simulink model "clearing_faulted_segment_travelling_Wave"  (R2018a)
settings: Solver=ode23t  StartTime=0.0  StopTime=2  MaxStep=1e-3  RelTol=1e-3
values from neighbouring files (symbols this model uses):
  AC_lim = [1.5 -1.5]    [MT_HVDC_initialize.m]
  C_pm = 10.48e-3    (= 0.01048)    [MT_HVDC_initialize.m]
  ccsc_lim = [1.0 -1.0]    [MT_HVDC_initialize.m]
  DC_lim = [1.05 -1.05]    [MT_HVDC_initialize.m]
  f = 50    [MT_HVDC_initialize.m]
  Fc = 50    [MT_HVDC_initialize.m]
  Fn_filter = 1000    [MT_HVDC_initialize.m]
  Ireg_lim_i = [1.5, -1.5]    [MT_HVDC_initialize.m]
  Ireg_lim_r = [1.5, -1.5]    [MT_HVDC_initialize.m]
  Ki_ACreg_i = 260    [MT_HVDC_initialize.m]
  Ki_ccsc = 5    [MT_HVDC_initialize.m]
  Ki_DCreg_r = 150    [MT_HVDC_initialize.m]
  Ki_Ireg_i = 200    [MT_HVDC_initialize.m]
  Ki_Ireg_r = 100    [MT_HVDC_initialize.m]
  Ki_R_inv = 150000    [MT_HVDC_initialize.m]
  Ki_R_rec = 5000    [MT_HVDC_initialize.m]
  Kp_ACreg_i = 2    [MT_HVDC_initialize.m]
  Kp_ccsc = 1    [MT_HVDC_initialize.m]
  Kp_DCreg_r = 8    [MT_HVDC_initialize.m]
  Kp_Ireg_i = 2    [MT_HVDC_initialize.m]
  Kp_Ireg_r = 2    [MT_HVDC_initialize.m]
  Kp_R_inv = 0.001    [MT_HVDC_initialize.m]
  Kp_R_rec = 0.001    [MT_HVDC_initialize.m]
  L1_pu = 0.109    [MT_HVDC_initialize.m]
  L2_pu = 0.0824    [MT_HVDC_initialize.m]
  L_arm = L_arm_pu*Z_base66/w    [MT_HVDC_initialize.m]
  L_arm_pu = 0.15    [MT_HVDC_initialize.m]
  L_int = X_int/w    [MT_HVDC_initialize.m]
  n = 50    [MT_HVDC_initialize.m]
  n2 = 50    [MT_HVDC_initialize.m]
  P_nom = 220e6    (= 220000000)    [MT_HVDC_initialize.m]
  R1_pu = 0.00206    [MT_HVDC_initialize.m]
  R2_pu = 0.00206    [MT_HVDC_initialize.m]
  R_arm = 0.03    [MT_HVDC_initialize.m]
  R_arm_pu = R_arm/Z_base66    [MT_HVDC_initialize.m]
  R_int = sqrt((z_int_400^2)/(1+xr_ratio^2))    [MT_HVDC_initialize.m]
  Rg_T1 = 40    [MT_HVDC_initialize.m]
  S1_nom = P_nom    (= 220000000)    [MT_HVDC_initialize.m]
  S2_nom = P_nom    (= 220000000)    [MT_HVDC_initialize.m]
  T_fault = 1.4    [MT_HVDC_initialize.m]
  Ts_Control = 40e-6    (= 4e-05)    [MT_HVDC_initialize.m]
  Ts_Power = 20e-6    (= 2e-05)    [MT_HVDC_initialize.m]
  V1_prim = V_prim    (= 400000)    [MT_HVDC_initialize.m]
  V1_sec = V_grid    (= 66000)    [MT_HVDC_initialize.m]
  V2_prim = V_grid    (= 66000)    [MT_HVDC_initialize.m]
  V2_sec = 18e3    (= 18000)    [MT_HVDC_initialize.m]
  V_ac_ref = 1.035    [MT_HVDC_initialize.m]
  V_grid = 66e3    (= 66000)    [MT_HVDC_initialize.m]
  V_prim = 400e3    (= 400000)    [MT_HVDC_initialize.m]
  Vc_pm_r = 0*Vdc_nom/n    (= 0)    [MT_HVDC_initialize.m]
  Vdc_nom = 135e3    (= 135000)    [MT_HVDC_initialize.m]
  w = 2*pi*f    (= 314.159265359)    [MT_HVDC_initialize.m]
  z0z1 = 0.8    [MT_HVDC_initialize.m]
  Zeta_filter = 1    [MT_HVDC_initialize.m]
undefined symbols (not defined in the file or in its folder): D1, Delta, DiscIntNeverNeededParam
libraries: powerlib x417, powerlib_meascontrol x130, simulink x84, powerlib_extras x8, simulink_extras x5
(part 3 of 17)

== system clearing_faulted_segment_travelling_Wave/MMC Converter1 ==
  g : Inport
  Current Measurement{,1..5} (6 alike) : powerlib/Measurements/Current Measurement  PhasorSimulation=off  OutputType=Complex  PSBequivalent=0
      settings: SourceProductName=Simscape Electrical
  Demux : Demux  Outputs=6
  Half-Bridge MMC Ap : Subsystem  mask(Half-Bridge MMC - Aggregate Model){n=n, C=C_pm, Vc_Initial=Vc_pm_r, Ts=Ts_Power}
      mask prompts: n "Number of power modules"; C "Capacitor value (F):"; Vc_Initial "Capacitor initial voltage (V):"; Ts "Sample time (s):"
      mask help:
      | Implement a half-bridge Modular Multilevel Converter (MMC) using a switching-function model where only one equivalent module is used to represent all power modules.
      |
      | The control signal is a two-element vector [ Nin, Nbl ], where Nin represents the number of inserted modules and Nbl represents the number of modules in the blocked-state. The output Vc (capacitor voltage) has only one element and gives the average value of the capacitors modules.
      |
      | With this aggregate model, it is assumed that capacitor voltage of all power modules are well-balanced. However, control system dynamics, converter harmonics content and circulating currents phenomena are all-well represented. The model runs a lot faster than the detailed model which uses two switching devices and one capacitor for each individual power module. This aggregate model is also well-suited for real-time simulation.
      settings: AttributesFormatString=(Aggregate model of %<n> PM)
      mask Display:
      | x1=0.0;
      | plot([0.17 0.5]+x1,[0.93 0.93])
      | plot([0.5 0.5]+x1,[0.93,0.80])
      | plot([0.5 0.38]+x1,[0.80 0.74])
      | plot([0.38 0.38]+x1,[0.80 0.62])
      | plot([0.38 0.5]+x1,[0.68 0.62])
      | plot([0.5 0.5]+x1,[0.62 0.52])
      | plot([0.45 0.5 0.43]+x1,[0.68 0.62 0.60])
      | %
      | y1=0.40-0.03;
      | plot([0.5 0.5]+x1,[0.93,0.80]-y1)
      | plot([0.5 0.38]+x1,[0.80 0.74]-y1)
      | plot([0.38 0.38]+x1,[0.80 0.62]-y1)
      | plot([0.38 0.5]+x1,[0.68 0.62]-y1)
      | plot([0.5 0.5]+x1,[0.62 0.52]-y1)
      | plot([0.45 0.5 0.43]+x1,[0.68 0.62 0.60]-y1)
      | plot([0.5 0.5]+x1,[0.2,0.10])
      | plot([0.17 0.5]+x1,[0.1 0.1])
      | %
      | plot([0.5 0.6]+x1,[0.84 0.84]+0.03)
      | plot([0.6 0.6]+x1,[0.84 0.74]+0.03)
      | plot([0.6 0.56]+x1,[0.74 0.69]+0.03)
      | plot([0.6 0.64]+x1,[0.74 0.69]+0.03)
      | plot([0.56 0.64]+x1,[0.69 0.69]+0.03)
      | plot([0.6 0.6]+x1,[0.69 0.57]+0.03)
      | plot([0.5 0.6]+x1,[0.57 0.57]+0.03)
      | plot([0.55 0.65]+x1,[0.74 0.74]+0.03)
      | %
      | y2=0.4-0.03;
      | plot([0.5 0.6]+x1,[0.84 0.84]-y2)
      | plot([0.6 0.6]+x1,[0.84 0.74]-y2)
      | plot([0.6 0.56]+x1,[0.74 0.69]-y2)
      | plot([0.6 0.64]+x1,[0.74 0.69]-y2)
      | plot([0.56 0.64]+x1,[0.69 0.69]-y2)
      | plot([0.6 0.6]+x1,[0.69 0.57]-y2)
      | plot([0.5 0.6]+x1,[0.57 0.57]-y2)
      | plot([0.55 0.65]+x1,[0.74 0.74]-y2)
      | %
      | plot([0.5 0.75]+x1,[0.53 0.53])
      | plot([0.75 0.75]+x1,[0.53 0.57])
      | plot([0.75 0.75]+x1,[0.61 0.65])
      | plot([0.75 0.75]+x1,[0.69 0.73])
      | plot([0.75 0.75]+x1,[0.77 0.81])
      | plot([0.75 0.75]+x1,[0.09 0.07])
      | plot([0.75 0.75]+x1,[0.04 0.01])
      | %
      | plot([0.34 0.34]+x1,[0.65 0.75])
      | plot([0.28 0.34]+x1,[0.7 0.7])
      | %
      | plot([0.34 0.34]+x1,[0.65 0.75]-y2)
      | plot([0.28 0.34]+x1,[0.7 0.7]-y2)
      | %
      | %Capacitor
      | plot([0.16 0.16],[0.93 0.54])
      | plot([0.16 0.16],[0.47 0.10])
      | plot([0.04 0.27],[0.54 0.54])
      | plot([0.04 0.27],[0.47 0.47])
      | %
      | plot([0.5 0.75],[0.1 0.1])
      | % text(0.78,0.5,'1')
      | % text(0.78,0.12,'2')
      | %
      | color('blue')
      | port_label('input',1,'N')
  Half-Bridge MMC Ap1 : Subsystem  mask(Half-Bridge MMC - Aggregate Model){n=n, C=C_pm, Vc_Initial=Vc_pm_r, Ts=Ts_Power}
      mask prompts: n "Number of power modules"; C "Capacitor value (F):"; Vc_Initial "Capacitor initial voltage (V):"; Ts "Sample time (s):"
      mask help:
      | Implement a half-bridge Modular Multilevel Converter (MMC) using a switching-function model where only one equivalent module is used to represent all power modules.
      |
      | The control signal is a two-element vector [ Nin, Nbl ], where Nin represents the number of inserted modules and Nbl represents the number of modules in the blocked-state. The output Vc (capacitor voltage) has only one element and gives the average value of the capacitors modules.
      |
      | With this aggregate model, it is assumed that capacitor voltage of all power modules are well-balanced. However, control system dynamics, converter harmonics content and circulating currents phenomena are all-well represented. The model runs a lot faster than the detailed model which uses two switching devices and one capacitor for each individual power module. This aggregate model is also well-suited for real-time simulation.
      settings: AttributesFormatString=(Aggregate model of %<n> PM)
      mask Display:
      | x1=0.0;
      | plot([0.17 0.5]+x1,[0.93 0.93])
      | plot([0.5 0.5]+x1,[0.93,0.80])
      | plot([0.5 0.38]+x1,[0.80 0.74])
      | plot([0.38 0.38]+x1,[0.80 0.62])
      | plot([0.38 0.5]+x1,[0.68 0.62])
      | plot([0.5 0.5]+x1,[0.62 0.52])
      | plot([0.45 0.5 0.43]+x1,[0.68 0.62 0.60])
      | %
      | y1=0.40-0.03;
      | plot([0.5 0.5]+x1,[0.93,0.80]-y1)
      | plot([0.5 0.38]+x1,[0.80 0.74]-y1)
      | plot([0.38 0.38]+x1,[0.80 0.62]-y1)
      | plot([0.38 0.5]+x1,[0.68 0.62]-y1)
      | plot([0.5 0.5]+x1,[0.62 0.52]-y1)
      | plot([0.45 0.5 0.43]+x1,[0.68 0.62 0.60]-y1)
      | plot([0.5 0.5]+x1,[0.2,0.10])
      | plot([0.17 0.5]+x1,[0.1 0.1])
      | %
      | plot([0.5 0.6]+x1,[0.84 0.84]+0.03)
      | plot([0.6 0.6]+x1,[0.84 0.74]+0.03)
      | plot([0.6 0.56]+x1,[0.74 0.69]+0.03)
      | plot([0.6 0.64]+x1,[0.74 0.69]+0.03)
      | plot([0.56 0.64]+x1,[0.69 0.69]+0.03)
      | plot([0.6 0.6]+x1,[0.69 0.57]+0.03)
      | plot([0.5 0.6]+x1,[0.57 0.57]+0.03)
      | plot([0.55 0.65]+x1,[0.74 0.74]+0.03)
      | %
      | y2=0.4-0.03;
      | plot([0.5 0.6]+x1,[0.84 0.84]-y2)
      | plot([0.6 0.6]+x1,[0.84 0.74]-y2)
      | plot([0.6 0.56]+x1,[0.74 0.69]-y2)
      | plot([0.6 0.64]+x1,[0.74 0.69]-y2)
      | plot([0.56 0.64]+x1,[0.69 0.69]-y2)
      | plot([0.6 0.6]+x1,[0.69 0.57]-y2)
      | plot([0.5 0.6]+x1,[0.57 0.57]-y2)
      | plot([0.55 0.65]+x1,[0.74 0.74]-y2)
      | %
      | plot([0.5 0.75]+x1,[0.53 0.53])
      | plot([0.75 0.75]+x1,[0.53 0.57])
      | plot([0.75 0.75]+x1,[0.61 0.65])
      | plot([0.75 0.75]+x1,[0.69 0.73])
      | plot([0.75 0.75]+x1,[0.77 0.81])
      | plot([0.75 0.75]+x1,[0.09 0.07])
      | plot([0.75 0.75]+x1,[0.04 0.01])
      | %
      | plot([0.34 0.34]+x1,[0.65 0.75])
      | plot([0.28 0.34]+x1,[0.7 0.7])
      | %
      | plot([0.34 0.34]+x1,[0.65 0.75]-y2)
      | plot([0.28 0.34]+x1,[0.7 0.7]-y2)
      | %
      | %Capacitor
      | plot([0.16 0.16],[0.93 0.54])
      | plot([0.16 0.16],[0.47 0.10])
      | plot([0.04 0.27],[0.54 0.54])
      | plot([0.04 0.27],[0.47 0.47])
      | %
      | plot([0.5 0.75],[0.1 0.1])
      | % text(0.78,0.5,'1')
      | % text(0.78,0.12,'2')
      | %
      | color('blue')
      | port_label('input',1,'N')
  Half-Bridge MMC Ap2 : Subsystem  mask(Half-Bridge MMC - Aggregate Model){n=n, C=C_pm, Vc_Initial=Vc_pm_r, Ts=Ts_Power}
      mask prompts: n "Number of power modules"; C "Capacitor value (F):"; Vc_Initial "Capacitor initial voltage (V):"; Ts "Sample time (s):"
      mask help:
      | Implement a half-bridge Modular Multilevel Converter (MMC) using a switching-function model where only one equivalent module is used to represent all power modules.
      |
      | The control signal is a two-element vector [ Nin, Nbl ], where Nin represents the number of inserted modules and Nbl represents the number of modules in the blocked-state. The output Vc (capacitor voltage) has only one element and gives the average value of the capacitors modules.
      |
      | With this aggregate model, it is assumed that capacitor voltage of all power modules are well-balanced. However, control system dynamics, converter harmonics content and circulating currents phenomena are all-well represented. The model runs a lot faster than the detailed model which uses two switching devices and one capacitor for each individual power module. This aggregate model is also well-suited for real-time simulation.
      settings: AttributesFormatString=(Aggregate model of %<n> PM)
      mask Display:
      | x1=0.0;
      | plot([0.17 0.5]+x1,[0.93 0.93])
      | plot([0.5 0.5]+x1,[0.93,0.80])
      | plot([0.5 0.38]+x1,[0.80 0.74])
      | plot([0.38 0.38]+x1,[0.80 0.62])
      | plot([0.38 0.5]+x1,[0.68 0.62])
      | plot([0.5 0.5]+x1,[0.62 0.52])
      | plot([0.45 0.5 0.43]+x1,[0.68 0.62 0.60])
      | %
      | y1=0.40-0.03;
      | plot([0.5 0.5]+x1,[0.93,0.80]-y1)
      | plot([0.5 0.38]+x1,[0.80 0.74]-y1)
      | plot([0.38 0.38]+x1,[0.80 0.62]-y1)
      | plot([0.38 0.5]+x1,[0.68 0.62]-y1)
      | plot([0.5 0.5]+x1,[0.62 0.52]-y1)
      | plot([0.45 0.5 0.43]+x1,[0.68 0.62 0.60]-y1)
      | plot([0.5 0.5]+x1,[0.2,0.10])
      | plot([0.17 0.5]+x1,[0.1 0.1])
      | %
      | plot([0.5 0.6]+x1,[0.84 0.84]+0.03)
      | plot([0.6 0.6]+x1,[0.84 0.74]+0.03)
      | plot([0.6 0.56]+x1,[0.74 0.69]+0.03)
      | plot([0.6 0.64]+x1,[0.74 0.69]+0.03)
      | plot([0.56 0.64]+x1,[0.69 0.69]+0.03)
      | plot([0.6 0.6]+x1,[0.69 0.57]+0.03)
      | plot([0.5 0.6]+x1,[0.57 0.57]+0.03)
      | plot([0.55 0.65]+x1,[0.74 0.74]+0.03)
      | %
      | y2=0.4-0.03;
      | plot([0.5 0.6]+x1,[0.84 0.84]-y2)
      | plot([0.6 0.6]+x1,[0.84 0.74]-y2)
      | plot([0.6 0.56]+x1,[0.74 0.69]-y2)
      | plot([0.6 0.64]+x1,[0.74 0.69]-y2)
      | plot([0.56 0.64]+x1,[0.69 0.69]-y2)
      | plot([0.6 0.6]+x1,[0.69 0.57]-y2)
      | plot([0.5 0.6]+x1,[0.57 0.57]-y2)
      | plot([0.55 0.65]+x1,[0.74 0.74]-y2)
      | %
      | plot([0.5 0.75]+x1,[0.53 0.53])
      | plot([0.75 0.75]+x1,[0.53 0.57])
      | plot([0.75 0.75]+x1,[0.61 0.65])
      | plot([0.75 0.75]+x1,[0.69 0.73])
      | plot([0.75 0.75]+x1,[0.77 0.81])
      | plot([0.75 0.75]+x1,[0.09 0.07])
      | plot([0.75 0.75]+x1,[0.04 0.01])
      | %
      | plot([0.34 0.34]+x1,[0.65 0.75])
      | plot([0.28 0.34]+x1,[0.7 0.7])
      | %
      | plot([0.34 0.34]+x1,[0.65 0.75]-y2)
      | plot([0.28 0.34]+x1,[0.7 0.7]-y2)
      | %
      | %Capacitor
      | plot([0.16 0.16],[0.93 0.54])
      | plot([0.16 0.16],[0.47 0.10])
      | plot([0.04 0.27],[0.54 0.54])
      | plot([0.04 0.27],[0.47 0.47])
      | %
      | plot([0.5 0.75],[0.1 0.1])
      | % text(0.78,0.5,'1')
      | % text(0.78,0.12,'2')
      | %
      | color('blue')
      | port_label('input',1,'N')
  Half-Bridge MMC Ap3 : Subsystem  mask(Half-Bridge MMC - Aggregate Model){n=n, C=C_pm, Vc_Initial=Vc_pm_r, Ts=Ts_Power}
      mask prompts: n "Number of power modules"; C "Capacitor value (F):"; Vc_Initial "Capacitor initial voltage (V):"; Ts "Sample time (s):"
      mask help:
      | Implement a half-bridge Modular Multilevel Converter (MMC) using a switching-function model where only one equivalent module is used to represent all power modules.
      |
      | The control signal is a two-element vector [ Nin, Nbl ], where Nin represents the number of inserted modules and Nbl represents the number of modules in the blocked-state. The output Vc (capacitor voltage) has only one element and gives the average value of the capacitors modules.
      |
      | With this aggregate model, it is assumed that capacitor voltage of all power modules are well-balanced. However, control system dynamics, converter harmonics content and circulating currents phenomena are all-well represented. The model runs a lot faster than the detailed model which uses two switching devices and one capacitor for each individual power module. This aggregate model is also well-suited for real-time simulation.
      settings: AttributesFormatString=(Aggregate model of %<n> PM)
      mask Display:
      | x1=0.0;
      | plot([0.17 0.5]+x1,[0.93 0.93])
      | plot([0.5 0.5]+x1,[0.93,0.80])
      | plot([0.5 0.38]+x1,[0.80 0.74])
      | plot([0.38 0.38]+x1,[0.80 0.62])
      | plot([0.38 0.5]+x1,[0.68 0.62])
      | plot([0.5 0.5]+x1,[0.62 0.52])
      | plot([0.45 0.5 0.43]+x1,[0.68 0.62 0.60])
      | %
      | y1=0.40-0.03;
      | plot([0.5 0.5]+x1,[0.93,0.80]-y1)
      | plot([0.5 0.38]+x1,[0.80 0.74]-y1)
      | plot([0.38 0.38]+x1,[0.80 0.62]-y1)
      | plot([0.38 0.5]+x1,[0.68 0.62]-y1)
      | plot([0.5 0.5]+x1,[0.62 0.52]-y1)
      | plot([0.45 0.5 0.43]+x1,[0.68 0.62 0.60]-y1)
      | plot([0.5 0.5]+x1,[0.2,0.10])
      | plot([0.17 0.5]+x1,[0.1 0.1])
      | %
      | plot([0.5 0.6]+x1,[0.84 0.84]+0.03)
      | plot([0.6 0.6]+x1,[0.84 0.74]+0.03)
      | plot([0.6 0.56]+x1,[0.74 0.69]+0.03)
      | plot([0.6 0.64]+x1,[0.74 0.69]+0.03)
      | plot([0.56 0.64]+x1,[0.69 0.69]+0.03)
      | plot([0.6 0.6]+x1,[0.69 0.57]+0.03)
      | plot([0.5 0.6]+x1,[0.57 0.57]+0.03)
      | plot([0.55 0.65]+x1,[0.74 0.74]+0.03)
      | %
      | y2=0.4-0.03;
      | plot([0.5 0.6]+x1,[0.84 0.84]-y2)
      | plot([0.6 0.6]+x1,[0.84 0.74]-y2)
      | plot([0.6 0.56]+x1,[0.74 0.69]-y2)
      | plot([0.6 0.64]+x1,[0.74 0.69]-y2)
      | plot([0.56 0.64]+x1,[0.69 0.69]-y2)
      | plot([0.6 0.6]+x1,[0.69 0.57]-y2)
      | plot([0.5 0.6]+x1,[0.57 0.57]-y2)
      | plot([0.55 0.65]+x1,[0.74 0.74]-y2)
      | %
      | plot([0.5 0.75]+x1,[0.53 0.53])
      | plot([0.75 0.75]+x1,[0.53 0.57])
      | plot([0.75 0.75]+x1,[0.61 0.65])
      | plot([0.75 0.75]+x1,[0.69 0.73])
      | plot([0.75 0.75]+x1,[0.77 0.81])
      | plot([0.75 0.75]+x1,[0.09 0.07])
      | plot([0.75 0.75]+x1,[0.04 0.01])
      | %
      | plot([0.34 0.34]+x1,[0.65 0.75])
      | plot([0.28 0.34]+x1,[0.7 0.7])
      | %
      | plot([0.34 0.34]+x1,[0.65 0.75]-y2)
      | plot([0.28 0.34]+x1,[0.7 0.7]-y2)
      | %
      | %Capacitor
      | plot([0.16 0.16],[0.93 0.54])
      | plot([0.16 0.16],[0.47 0.10])
      | plot([0.04 0.27],[0.54 0.54])
      | plot([0.04 0.27],[0.47 0.47])
      | %
      | plot([0.5 0.75],[0.1 0.1])
      | % text(0.78,0.5,'1')
      | % text(0.78,0.12,'2')
      | %
      | color('blue')
      | port_label('input',1,'N')
  Half-Bridge MMC Ap4 : Subsystem  mask(Half-Bridge MMC - Aggregate Model){n=n, C=C_pm, Vc_Initial=Vc_pm_r, Ts=Ts_Power}
      mask prompts: n "Number of power modules"; C "Capacitor value (F):"; Vc_Initial "Capacitor initial voltage (V):"; Ts "Sample time (s):"
      mask help:
      | Implement a half-bridge Modular Multilevel Converter (MMC) using a switching-function model where only one equivalent module is used to represent all power modules.
      |
      | The control signal is a two-element vector [ Nin, Nbl ], where Nin represents the number of inserted modules and Nbl represents the number of modules in the blocked-state. The output Vc (capacitor voltage) has only one element and gives the average value of the capacitors modules.
      |
      | With this aggregate model, it is assumed that capacitor voltage of all power modules are well-balanced. However, control system dynamics, converter harmonics content and circulating currents phenomena are all-well represented. The model runs a lot faster than the detailed model which uses two switching devices and one capacitor for each individual power module. This aggregate model is also well-suited for real-time simulation.
      settings: AttributesFormatString=(Aggregate model of %<n> PM)
      mask Display:
      | x1=0.0;
      | plot([0.17 0.5]+x1,[0.93 0.93])
      | plot([0.5 0.5]+x1,[0.93,0.80])
      | plot([0.5 0.38]+x1,[0.80 0.74])
      | plot([0.38 0.38]+x1,[0.80 0.62])
      | plot([0.38 0.5]+x1,[0.68 0.62])
      | plot([0.5 0.5]+x1,[0.62 0.52])
      | plot([0.45 0.5 0.43]+x1,[0.68 0.62 0.60])
      | %
      | y1=0.40-0.03;
      | plot([0.5 0.5]+x1,[0.93,0.80]-y1)
      | plot([0.5 0.38]+x1,[0.80 0.74]-y1)
      | plot([0.38 0.38]+x1,[0.80 0.62]-y1)
      | plot([0.38 0.5]+x1,[0.68 0.62]-y1)
      | plot([0.5 0.5]+x1,[0.62 0.52]-y1)
      | plot([0.45 0.5 0.43]+x1,[0.68 0.62 0.60]-y1)
      | plot([0.5 0.5]+x1,[0.2,0.10])
      | plot([0.17 0.5]+x1,[0.1 0.1])
      | %
      | plot([0.5 0.6]+x1,[0.84 0.84]+0.03)
      | plot([0.6 0.6]+x1,[0.84 0.74]+0.03)
      | plot([0.6 0.56]+x1,[0.74 0.69]+0.03)
      | plot([0.6 0.64]+x1,[0.74 0.69]+0.03)
      | plot([0.56 0.64]+x1,[0.69 0.69]+0.03)
      | plot([0.6 0.6]+x1,[0.69 0.57]+0.03)
      | plot([0.5 0.6]+x1,[0.57 0.57]+0.03)
      | plot([0.55 0.65]+x1,[0.74 0.74]+0.03)
      | %
      | y2=0.4-0.03;
      | plot([0.5 0.6]+x1,[0.84 0.84]-y2)
      | plot([0.6 0.6]+x1,[0.84 0.74]-y2)
      | plot([0.6 0.56]+x1,[0.74 0.69]-y2)
      | plot([0.6 0.64]+x1,[0.74 0.69]-y2)
      | plot([0.56 0.64]+x1,[0.69 0.69]-y2)
      | plot([0.6 0.6]+x1,[0.69 0.57]-y2)
      | plot([0.5 0.6]+x1,[0.57 0.57]-y2)
      | plot([0.55 0.65]+x1,[0.74 0.74]-y2)
      | %
      | plot([0.5 0.75]+x1,[0.53 0.53])
      | plot([0.75 0.75]+x1,[0.53 0.57])
      | plot([0.75 0.75]+x1,[0.61 0.65])
      | plot([0.75 0.75]+x1,[0.69 0.73])
      | plot([0.75 0.75]+x1,[0.77 0.81])
      | plot([0.75 0.75]+x1,[0.09 0.07])
      | plot([0.75 0.75]+x1,[0.04 0.01])
      | %
      | plot([0.34 0.34]+x1,[0.65 0.75])
      | plot([0.28 0.34]+x1,[0.7 0.7])
      | %
      | plot([0.34 0.34]+x1,[0.65 0.75]-y2)
      | plot([0.28 0.34]+x1,[0.7 0.7]-y2)
      | %
      | %Capacitor
      | plot([0.16 0.16],[0.93 0.54])
      | plot([0.16 0.16],[0.47 0.10])
      | plot([0.04 0.27],[0.54 0.54])
      | plot([0.04 0.27],[0.47 0.47])
      | %
      | plot([0.5 0.75],[0.1 0.1])
      | % text(0.78,0.5,'1')
      | % text(0.78,0.12,'2')
      | %
      | color('blue')
      | port_label('input',1,'N')
  Half-Bridge MMC Ap5 : Subsystem  mask(Half-Bridge MMC - Aggregate Model){n=n, C=C_pm, Vc_Initial=Vc_pm_r, Ts=Ts_Power}
      mask prompts: n "Number of power modules"; C "Capacitor value (F):"; Vc_Initial "Capacitor initial voltage (V):"; Ts "Sample time (s):"
      mask help:
      | Implement a half-bridge Modular Multilevel Converter (MMC) using a switching-function model where only one equivalent module is used to represent all power modules.
      |
      | The control signal is a two-element vector [ Nin, Nbl ], where Nin represents the number of inserted modules and Nbl represents the number of modules in the blocked-state. The output Vc (capacitor voltage) has only one element and gives the average value of the capacitors modules.
      |
      | With this aggregate model, it is assumed that capacitor voltage of all power modules are well-balanced. However, control system dynamics, converter harmonics content and circulating currents phenomena are all-well represented. The model runs a lot faster than the detailed model which uses two switching devices and one capacitor for each individual power module. This aggregate model is also well-suited for real-time simulation.
      settings: AttributesFormatString=(Aggregate model of %<n> PM)
      mask Display:
      | x1=0.0;
      | plot([0.17 0.5]+x1,[0.93 0.93])
      | plot([0.5 0.5]+x1,[0.93,0.80])
      | plot([0.5 0.38]+x1,[0.80 0.74])
      | plot([0.38 0.38]+x1,[0.80 0.62])
      | plot([0.38 0.5]+x1,[0.68 0.62])
      | plot([0.5 0.5]+x1,[0.62 0.52])
      | plot([0.45 0.5 0.43]+x1,[0.68 0.62 0.60])
      | %
      | y1=0.40-0.03;
      | plot([0.5 0.5]+x1,[0.93,0.80]-y1)
      | plot([0.5 0.38]+x1,[0.80 0.74]-y1)
      | plot([0.38 0.38]+x1,[0.80 0.62]-y1)
      | plot([0.38 0.5]+x1,[0.68 0.62]-y1)
      | plot([0.5 0.5]+x1,[0.62 0.52]-y1)
      | plot([0.45 0.5 0.43]+x1,[0.68 0.62 0.60]-y1)
      | plot([0.5 0.5]+x1,[0.2,0.10])
      | plot([0.17 0.5]+x1,[0.1 0.1])
      | %
      | plot([0.5 0.6]+x1,[0.84 0.84]+0.03)
      | plot([0.6 0.6]+x1,[0.84 0.74]+0.03)
      | plot([0.6 0.56]+x1,[0.74 0.69]+0.03)
      | plot([0.6 0.64]+x1,[0.74 0.69]+0.03)
      | plot([0.56 0.64]+x1,[0.69 0.69]+0.03)
      | plot([0.6 0.6]+x1,[0.69 0.57]+0.03)
      | plot([0.5 0.6]+x1,[0.57 0.57]+0.03)
      | plot([0.55 0.65]+x1,[0.74 0.74]+0.03)
      | %
      | y2=0.4-0.03;
      | plot([0.5 0.6]+x1,[0.84 0.84]-y2)
      | plot([0.6 0.6]+x1,[0.84 0.74]-y2)
      | plot([0.6 0.56]+x1,[0.74 0.69]-y2)
      | plot([0.6 0.64]+x1,[0.74 0.69]-y2)
      | plot([0.56 0.64]+x1,[0.69 0.69]-y2)
      | plot([0.6 0.6]+x1,[0.69 0.57]-y2)
      | plot([0.5 0.6]+x1,[0.57 0.57]-y2)
      | plot([0.55 0.65]+x1,[0.74 0.74]-y2)
      | %
      | plot([0.5 0.75]+x1,[0.53 0.53])
      | plot([0.75 0.75]+x1,[0.53 0.57])
      | plot([0.75 0.75]+x1,[0.61 0.65])
      | plot([0.75 0.75]+x1,[0.69 0.73])
      | plot([0.75 0.75]+x1,[0.77 0.81])
      | plot([0.75 0.75]+x1,[0.09 0.07])
      | plot([0.75 0.75]+x1,[0.04 0.01])
      | %
      | plot([0.34 0.34]+x1,[0.65 0.75])
      | plot([0.28 0.34]+x1,[0.7 0.7])
      | %
      | plot([0.34 0.34]+x1,[0.65 0.75]-y2)
      | plot([0.28 0.34]+x1,[0.7 0.7]-y2)
      | %
      | %Capacitor
      | plot([0.16 0.16],[0.93 0.54])
      | plot([0.16 0.16],[0.47 0.10])
      | plot([0.04 0.27],[0.54 0.54])
      | plot([0.04 0.27],[0.47 0.47])
      | %
      | plot([0.5 0.75],[0.1 0.1])
      | % text(0.78,0.5,'1')
      | % text(0.78,0.12,'2')
      | %
      | color('blue')
      | port_label('input',1,'N')
  Mux : Mux  Inputs=6
  Mux1 : Mux  Inputs=6
  Series RLC Branch1 : powerlib/Elements/Series RLC Branch  LConnTagsString=__new0  RConnTagsString=__new0  BranchType=L  Resistance=R_arm  Inductance=L_arm  SetiL0=off  InitialCurrent=0  Capacitance=1e-6  Setx0=off  InitialVoltage=0  Measurements=None
      settings: SourceProductName=Simscape Electrical
  Series RLC Branch{2..6} (5 alike) : powerlib/Elements/Series RLC Branch  LConnTagsString=__new0  RConnTagsString=__new0  BranchType=RL  Resistance=R_arm  Inductance=L_arm  SetiL0=off  InitialCurrent=0  Capacitance=1e-6  Setx0=off  InitialVoltage=0  Measurements=None
      settings: SourceProductName=Simscape Electrical
  Series RLC Branch7 : powerlib/Elements/Series RLC Branch  LConnTagsString=__new0  RConnTagsString=__new0  BranchType=R  Resistance=R_arm  Inductance=L_arm  SetiL0=off  InitialCurrent=0  Capacitance=1e-6  Setx0=off  InitialVoltage=0  Measurements=None
      settings: SourceProductName=Simscape Electrical
  V_a : PMIOPort  Tag=PMCPort  Side=Left
  V_b : PMIOPort  Tag=PMCPort  Port=2  Side=Left
  V_c : PMIOPort  Tag=PMCPort  Port=3  Side=Left
  Vdc + : PMIOPort  Tag=PMCPort  Port=4  Side=Right
  Vdc - : PMIOPort  Tag=PMCPort  Port=5  Side=Right
  Vc : Outport
  I_arm : Outport  Port=2
  wires:
  Demux/6 -> [g6]
  Demux/5 -> [g5]
  Demux/4 -> [g4]
  Demux/3 -> [g3]
  Demux/2 -> [g2]
  Demux/1 -> [g1]
  Half-Bridge MMC Ap/1(Vc) -> [Vc1]
  Half-Bridge MMC Ap5/1(Vc) -> [Vc6]
  Half-Bridge MMC Ap3/1(Vc) -> [Vc2]
  Half-Bridge MMC Ap4/1(Vc) -> [Vc5]
  [Icu] -> Mux1/5
  [Ibl] -> Mux1/4
  [Icl] -> Mux1/6
  [Ial] -> Mux1/2
  [Iau] -> Mux1/1
  Mux1/1 -> I_arm/1
  [Ibu] -> Mux1/3
  Current Measurement2/1 -> [Ibu]
  Current Measurement5/1 -> [Icl]
  Current Measurement3/1 -> [Icu]
  Current Measurement4/1 -> [Ibl]
  Current Measurement/1 -> [Iau]
  Current Measurement1/1 -> [Ial]
  [Vc5] -> Mux/5
  Mux/1 -> Vc/1
  [Vc4] -> Mux/4
  [Vc1] -> Mux/1
  [Vc6] -> Mux/6
  [Vc3] -> Mux/3
  [g5] -> Half-Bridge MMC Ap1/1(g)
  [g1] -> Half-Bridge MMC Ap/1(g)
  [g4] -> Half-Bridge MMC Ap3/1(g)
  [g3] -> Half-Bridge MMC Ap4/1(g)
  [g2] -> Half-Bridge MMC Ap2/1(g)
  [g6] -> Half-Bridge MMC Ap5/1(g)
  g/1 -> Demux/1
  [Vc2] -> Mux/2
  Half-Bridge MMC Ap1/1(Vc) -> [Vc4]
  Half-Bridge MMC Ap2/1(Vc) -> [Vc3]
  connections:
  Half-Bridge MMC Ap1/LConn1 -- Current Measurement4/RConn1
  Half-Bridge MMC Ap5/LConn1 -- Current Measurement5/RConn1
  Half-Bridge MMC Ap2/LConn2 -- Current Measurement2/LConn1
  Half-Bridge MMC Ap4/LConn2 -- Current Measurement3/LConn1
  Vdc -/RConn1 -- Half-Bridge MMC Ap3/LConn2 -- Half-Bridge MMC Ap5/LConn2 -- Half-Bridge MMC Ap1/LConn2
  Half-Bridge MMC Ap3/LConn1 -- Current Measurement1/RConn1
  V_b/RConn1 -- Series RLC Branch2/RConn1 -- Series RLC Branch4/LConn1
  Series RLC Branch1/LConn1 -- Series RLC Branch7/RConn1
  Series RLC Branch3/RConn1 -- Current Measurement1/LConn1
  V_c/RConn1 -- Series RLC Branch5/LConn1 -- Series RLC Branch6/RConn1
  V_a/RConn1 -- Series RLC Branch1/RConn1 -- Series RLC Branch3/LConn1
  Series RLC Branch2/LConn1 -- Current Measurement2/RConn1
  Series RLC Branch4/RConn1 -- Current Measurement4/LConn1
  Current Measurement5/LConn1 -- Series RLC Branch5/RConn1
  Series RLC Branch6/LConn1 -- Current Measurement3/RConn1
  Vdc +/RConn1 -- Half-Bridge MMC Ap/LConn1 -- Half-Bridge MMC Ap4/LConn1 -- Half-Bridge MMC Ap2/LConn1
  Current Measurement/LConn1 -- Half-Bridge MMC Ap/LConn2
  Series RLC Branch7/LConn1 -- Current Measurement/RConn1
